simulink subsystem "OpenDifferential2"  (R2025b)
settings: Solver=VariableStepAuto  StartTime=0.0  StopTime=10.0  RelTol=1e-3
libraries: autolibshareddiff x1
settings Model: Creator=The MathWorks, Inc.  LastModifiedBy=The MathWorks, Inc.
settings RTWCC: GPUComputeCapability=3.5

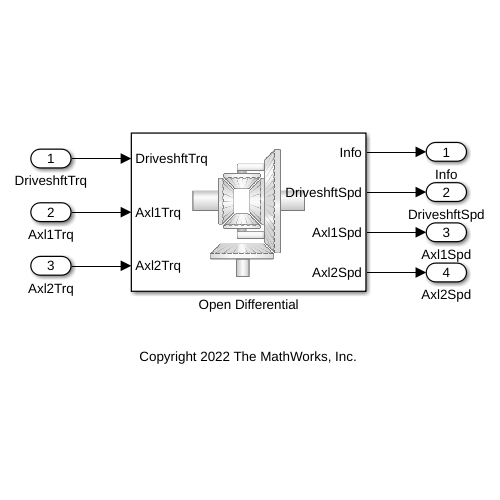
[thumbnail: Simulink's stored preview of the top-level diagram]
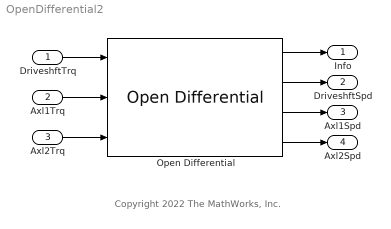
== system OpenDifferential2 ==
  note: Copyright 2022 The MathWorks, Inc.
  DriveshftTrq : Inport
  Axl1Trq : Inport  Port=2
  Axl2Trq : Inport  Port=3
  Open Differential : autolibshareddiff/Open Differential  VariantControl=Open Differential  DiffEffModelPopup=Constant  InterpMethod=Linear point-slope  extTamb=off  shaftSwitchMask=To the left of center-line  Ndiff=PlntDiffrntl2Ratio  Jd=PlntDiffrntl2CarrInertia  bd=PlntDiffrntl2CarrDamp  Jw1=PlntDiffrntl2Axl1Inertia  bw1=PlntDiffrntl2Axl1Damp  Jw2=PlntDiffrntl2Axl2Inertia  bw2=PlntDiffrntl2Axl2Damp  omegaw1o=PlntDiffrntl2Axl1InitVel  omegaw2o=PlntDiffrntl2Axl2InitVel  eta=PlntDiffrntl2Eff  eta_tbl=PlntDiffrntl2EffTbl  Trq_bpts=PlntDiffrntl2EffTrqBpt  omega_bpts=PlntDiffrntl2EffSpdBpt  Temp_bpts=PlntDiffrntl2EffTempBpt  Tamb=EnvAirTemp  maxAbsSpd=5e3  aMode=6
  Info : Outport
  DriveshftSpd : Outport  Port=2
  Axl1Spd : Outport  Port=3
  Axl2Spd : Outport  Port=4
  wires:
  Open Differential/1 -> Info/1
  Open Differential/2 -> DriveshftSpd/1
  Open Differential/3 -> Axl1Spd/1
  Open Differential/4 -> Axl2Spd/1
  DriveshftTrq/1 -> Open Differential/1
  Axl1Trq/1 -> Open Differential/2
  Axl2Trq/1 -> Open Differential/3
